simulink model "chap7_13sim"  (Simulink 3.00)
settings: Solver=ode45  StartTime=0.0  StopTime=20  RelTol=1e-3
values from neighbouring files (symbols this model uses):
  A = [0,1,0,0 ... (first row only)    [chap7_12.m]    (also in chap7_13.m = [ 0    1.0000         0         0         0         0)
  B = [0;t3;0;t4]    [chap7_12.m]    (also in chap7_13.m = [0; 9.48888; 0; 46.275; 0; -46.275])
  C = [1,0,0,0 ... (first row only)    [chap7_12.m]    (also in chap7_13.m = [1 0 0 0 0 0)
  D = [0;0]    [chap7_12.m]    (also in chap7_13.m = [0 0 0 0 0 0 ]')

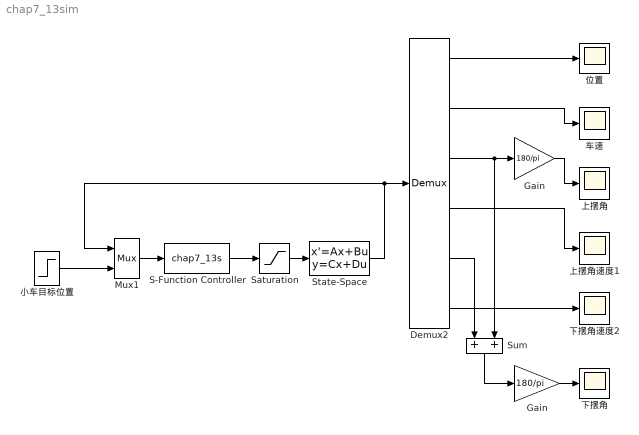
== system chap7_13sim ==
  Demux2 : Demux  Outputs=6
  Gain : Gain  Gain=180/pi  SaturateOnIntegerOverflow=on
  "Gain " : Gain  Gain=180/pi  SaturateOnIntegerOverflow=on
  Mux1 : Mux  Inputs=2
      settings: DisplayOption=none
  S-Function Controller : S-Function  FunctionName=chap7_13s  PortCounts=[]  SFunctionModules=''
  "Saturation " : Saturate  UpperLimit=5  LowerLimit=-5
  State-Space : StateSpace  A=A  B=B  C=C  D=D  X0=[0 0 1.2 0 -1.2 0 ]
  Sum : Sum  Orientation=down  Inputs=+|+  SaturateOnIntegerOverflow=on
  车速 : Scope
      settings: TimeRange=auto  YMin=-0.0011  YMax=-0.0001  SaveToWorkspace=off  SaveName=ScopeData  MaxRows=50000
  上摆角 : Scope
      settings: TimeRange=auto  YMin=-1  YMax=6  SaveToWorkspace=off  SaveName=ScopeData  MaxRows=50000
  上摆角速度1 : Scope
      settings: TimeRange=auto  YMin=-750  YMax=1000  SaveToWorkspace=off  SaveName=ScopeData  MaxRows=50000
  "位置  " : Scope
      settings: TimeRange=80  YMin=0.1  YMax=0.100006  SaveToWorkspace=off  SaveName=ScopeData  MaxRows=50000
  下摆角 : Scope
      settings: TimeRange=80  YMin=0  YMax=4e-006  SaveToWorkspace=off  SaveName=ScopeData  MaxRows=50000
  下摆角速度2 : Scope
      settings: TimeRange=auto  YMin=-35  YMax=35  SaveToWorkspace=off  SaveName=ScopeData  MaxRows=50000
  小车目标位置 : Step  Time=1  Before=0  After=0.1  SampleTime=0
  wires:
  Gain/1 -> 上摆角/1
  "Gain "/1 -> 下摆角/1
  Demux2/4 -> 上摆角速度1/1
  Demux2/6 -> 下摆角速度2/1
  Demux2/2 -> 车速/1
  Demux2/1 -> "位置  "/1
  State-Space/1 -> Demux2/1, Mux1/1
  S-Function Controller/1 -> "Saturation "/1
  "Saturation "/1 -> State-Space/1
  Mux1/1 -> S-Function Controller/1
  Sum/1 -> "Gain "/1
  小车目标位置/1 -> Mux1/2
  Demux2/5 -> Sum/1
  Demux2/3 -> Gain/1, Sum/2
